simulink model "Penduloinvertido_fcn"  (R2025a)
settings: Solver=VariableStepAuto  StartTime=0.0  StopTime=10.0  RelTol=1e-3
settings Model: Creator=azy51  LastModifiedBy=azy51

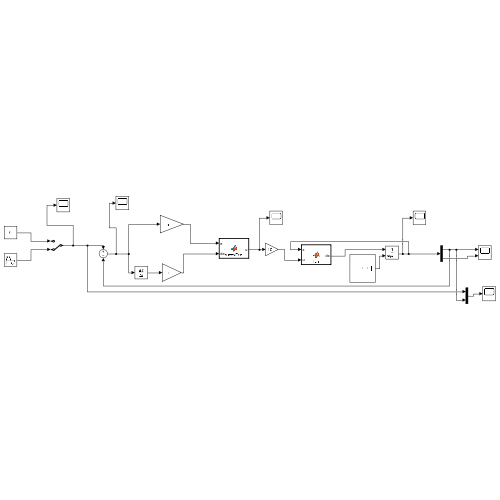
[thumbnail: Simulink's stored preview of the top-level diagram]
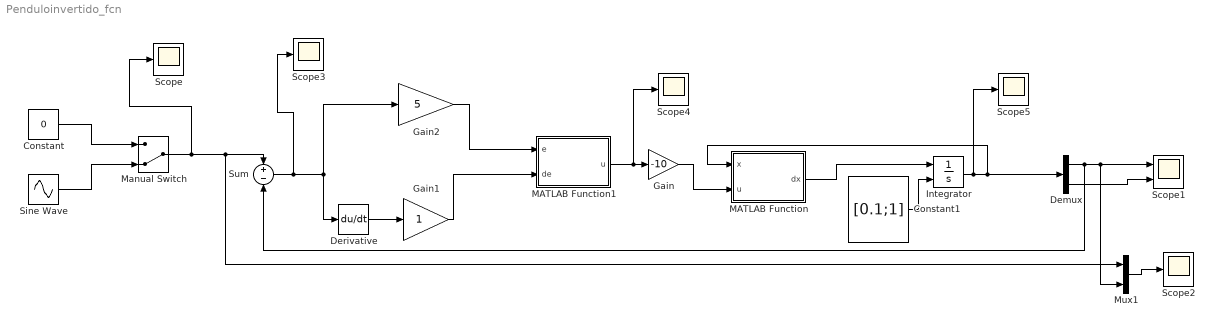
== system Penduloinvertido_fcn ==
  Constant : Constant  Value=0
  Constant1 : Constant  Value=[0.1;1]
  Demux : Demux  Outputs=2
  Derivative : Derivative
  Gain : Gain  Gain=-10
  Gain1 : Gain
  Gain2 : Gain  Gain=5
  Integrator : Integrator  InitialConditionSource=external
  MATLAB Function : MATLAB Function  TreatAsAtomicUnit=on
  MATLAB Function1 : MATLAB Function  TreatAsAtomicUnit=on
  Manual Switch : ManualSwitch  CurrentSetting=0
  Mux1 : Mux  Inputs=2
  Scope{,2..5} (5 alike) : Scope
      Scope settings: ActiveDisplayYMinimum=-1  ActiveDisplayYMaximum=1
      Scope2 settings: ActiveDisplayYMinimum=-1  ActiveDisplayYMaximum=1  DataLoggingVariableName=ScopeData2
      Scope3 settings: ActiveDisplayYMinimum=-1  ActiveDisplayYMaximum=1  DataLoggingVariableName=ScopeData3
      Scope4 settings: ActiveDisplayYMinimum=-1  ActiveDisplayYMaximum=1  DataLoggingVariableName=ScopeData4
      Scope5 settings: ActiveDisplayYMinimum=-1  ActiveDisplayYMaximum=1  DataLoggingVariableName=ScopeData5
  Scope1 : Scope  NumInputPorts=2
      settings: ActiveDisplayYMinimum=-5.7687864005876044  ActiveDisplayYMaximum=6.9848980239322236
  Sine Wave : Sin  Amplitude=.25  Frequency=4  SampleTime=0
  Sum : Sum  Inputs=+-
  wires:
  MATLAB Function1/1(u) -> Scope4/1, Gain/1
  Gain1/1 -> MATLAB Function1/2(de)
  Manual Switch/1 -> Scope/1, Mux1/1, Sum/1
  Demux/1 -> Sum/2, Mux1/2, Scope1/1
  Gain/1 -> MATLAB Function/2(u)
  Constant1/1 -> Integrator/2
  Mux1/1 -> Scope2/1
  Integrator/1 -> Scope5/1, Demux/1, MATLAB Function/1(x)
  Demux/2 -> Scope1/2
  Sine Wave/1 -> Manual Switch/2
  Derivative/1 -> Gain1/1
  MATLAB Function/1(dx) -> Integrator/1
  Constant/1 -> Manual Switch/1
  Sum/1 -> Scope3/1, Derivative/1, Gain2/1
  Gain2/1 -> MATLAB Function1/1(e)

== matlab function Penduloinvertido_fcn/MATLAB Function ==
  data: x input; dx output; u input
function dx  = fcn(x,u)

l=1; m=1; g=9.81; b=0.5; I=m*l^2;
x1=x(1);
x2=x(2);
dx1=x2;
dx2=g/l*sin(x1)-b*l/I*x2+u/I;
dx = [dx1;dx2];

== matlab function Penduloinvertido_fcn/MATLAB Function1 ==
  data: e input; u output; de input
function u = fuzzyFcn(e, de)
% Fuzzy Controller tipo Mamdani para péndulo invertido
% Entradas:
%   e  = error
%   de = delta error
% Salida:
%   u  = control

%% 1) Funciones de membresía de e
mu_e = zeros(5,1);
mu_e(1) = mf_trap(e, -pi, -pi, -pi/2, -pi/4); % e_nn
mu_e(2) = mf_tri(e, -pi/2, -pi/4, 0);         % e_n
mu_e(3) = mf_tri(e, -pi/4, 0, pi/4);          % e_z
mu_e(4) = mf_tri(e, 0, pi/4, pi/2);           % e_p
mu_e(5) = mf_trap(e, pi/4, pi/2, pi, pi);     % e_pp

%% 2) Funciones de membresía de de
mu_de = zeros(5,1);
mu_de(1) = mf_trap(de, -pi/2, -pi/2, -pi/4, -pi/8); % de_nn
mu_de(2) = mf_tri(de, -pi/4, -pi/8, 0);             % de_n
mu_de(3) = mf_tri(de, -pi/8, 0, pi/8);              % de_z
mu_de(4) = mf_tri(de, 0, pi/8, pi/4);               % de_p
mu_de(5) = mf_trap(de, pi/8, pi/4, pi/2, pi/2);     % de_pp

%% 3) Salidas fuzzy
u_range = -30:0.1:30;
u_mf = zeros(5,length(u_range));
u_mf(1,:) = mf_tri(u_range, -30, -20, -10); % u_nn
u_mf(2,:) = mf_tri(u_range, -20, -10, 0);   % u_n
u_mf(3,:) = mf_tri(u_range, -10, 0, 10);    % u_z
u_mf(4,:) = mf_tri(u_range, 0, 10, 20);     % u_p
u_mf(5,:) = mf_tri(u_range, 10, 20, 30);    % u_pp

%% 4) Reglas fuzzy en forma de matriz [salida_index]
% Filas: e_nn,e_n,e_z,e_p,e_pp
% Columnas: de_nn,de_n,de_z,de_p,de_pp
rule = [5 5 5 4 3;
        5 5 4 3 2;
        5 4 3 2 1;
        4 3 2 1 1;
        3 2 1 1 1];

%% 5) Inferencia
mu_out = zeros(1,length(u_range));
for i=1:5
    for j=1:5
        strength = min(mu_e(i), mu_de(j));
        mu_out = max(mu_out, strength * u_mf(rule(i,j),:));
    end
end

%% 6) Defuzzificación (centroide)
u = sum(u_range .* mu_out) / (sum(mu_out) + eps);

end

%% ===== Funciones auxiliares =====
function y = mf_trap(x,a,b,c,d)
if x <= a
    y = 0;
elseif x < b
    y = (x-a)/(b-a);
elseif x <= c
    y = 1;
elseif x < d
    y = (d-x)/(d-c);
else
    y = 0;
end
end

function y = mf_tri(x,a,b,c)
if x <= a
    y = 0;
elseif x <= b
    y = (x-a)/(b-a);
elseif x <= c
    y = (c-x)/(c-b);
else
    y = 0;
end
end
